simulink model "sg_lens_correct"  (Simulink 8.2)
settings: Solver=VariableStepDiscrete  StartTime=0.0  StopTime=7*Npxl  RelTol=1e-3
values from neighbouring files (symbols this model uses):
  ImgStrmIn = ImgDist'    [tb_lens_correct.m]
  ImgX = SizeI(2)    [tb_lens_correct.m]
  Npxl = ImgY * ImgX    [tb_lens_correct.m]
libraries: xbsIndex_r4 x10, dspsrcs4 x3
settings Model: Creator=sps  LastModifiedBy=tawassne
settings OptimizationCC: InitFltsAndDblsToZero=on
settings DebuggingCC: SaveWithParameterizedLinksMsg=none  SignalResolutionControl=TryResolveAllWithWarning  SolverPrmCheckMsg=none  MultiTaskDSMMsg=warning  MultiTaskCondExecSysMsg=none
settings RTWCC: IncludeERTFirstTime=on
settings GRTTargetCC: TargetFcnLib=ansi_tfl_tmw.mat

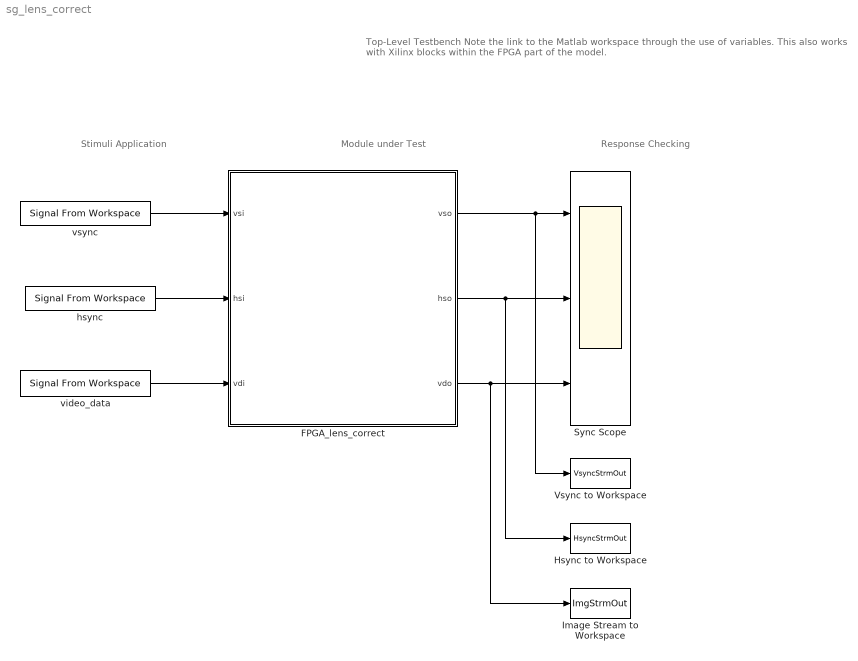
== system sg_lens_correct ==
  note: Top-Level Testbench
      | Note the link to the Matlab workspace through the use of variables.
      | This also works with Xilinx blocks within the FPGA part of the model.
  note: Stimuli Application
  note: Response Checking
  note: Module under Test
  FPGA_lens_correct : Subsystem
  Hsync to Workspace : ToWorkspace  VariableName=HsyncStrmOut  SampleTime=-1
      settings: MaxDataPoints=2*Npxl
  Image Stream to Workspace : ToWorkspace  VariableName=ImgStrmOut  SampleTime=-1
      settings: MaxDataPoints=2*Npxl
  Sync Scope : Scope  NumInputPorts=3
      settings: YMin=-5~-5~-5  YMax=5~5~5
  Vsync to Workspace : ToWorkspace  VariableName=VsyncStrmOut  SampleTime=-1
      settings: MaxDataPoints=2*Npxl
  hsync : dspsrcs4/Signal From Workspace  X=[ zeros(1,ImgX-1) 1 ]  Ts=1  nsamps=1  OutputAfterFinalValue=Cyclic repetition  ignoreOrWarnInputAndFrameLengths=off
  video_data : dspsrcs4/Signal From Workspace  X=[ ImgStrmIn(:) ]  Ts=1  nsamps=1  OutputAfterFinalValue=Cyclic repetition  ignoreOrWarnInputAndFrameLengths=off
  vsync : dspsrcs4/Signal From Workspace  X=[ zeros(1,Npxl-1) 1 ]  Ts=1  nsamps=1  OutputAfterFinalValue=Cyclic repetition  ignoreOrWarnInputAndFrameLengths=off
  wires:
  vsync/1 -> FPGA_lens_correct/1(vsi)
  hsync/1 -> FPGA_lens_correct/2(hsi)
  video_data/1 -> FPGA_lens_correct/3(vdi)
  FPGA_lens_correct/1(vso) -> Sync Scope/1, Vsync to Workspace/1
  FPGA_lens_correct/2(hso) -> Sync Scope/2, Hsync to Workspace/1
  FPGA_lens_correct/3(vdo) -> Sync Scope/3, Image Stream to Workspace/1

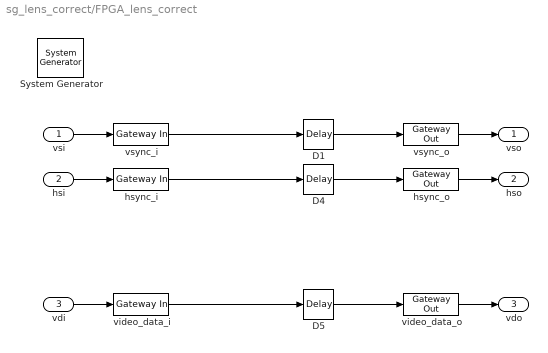
== system sg_lens_correct/FPGA_lens_correct ==
  vsi : Inport
  hsi : Inport  Port=2
  vdi : Inport  Port=3
  " System Generator" : xbsIndex_r4/ System Generator  Tag=genX  xilinxfamily=spartan6  part=xc6slx150t  speed=-3  package=fgg676  synthesis_tool=XST  clock_wrapper=Clock Enables  directory=./sg_gamma_s6  proj_type=Project Navigator  Synth_file=XST Defaults  Impl_file=ISE Defaults  testbench=off  simulink_period=1  sysclk_period=10  dcm_input_clock_period=10  incr_netlist=off  trim_vbits=Everywhere in SubSystem  dbl_ovrd=According to Block Masks  core_generation=According to Block Masks  run_coregen=off  deprecated_control=off  eval_field=0  block_type=sysgen
      settings: block_version=11.4
  D1 : xbsIndex_r4/Delay  rst=off  infoeditControl=Selection of Reset will increase slice count due to use of real FFs and instead of SRLs  en=off  latency=1  dbl_ovrd=off  reg_retiming=off  block_type=delay
  D4 : xbsIndex_r4/Delay  rst=off  infoeditControl=Selection of Reset will increase slice count due to use of real FFs and instead of SRLs  en=off  latency=1  dbl_ovrd=off  reg_retiming=off  block_type=delay
  D5 : xbsIndex_r4/Delay  rst=off  infoeditControl=Selection of Reset will increase slice count due to use of real FFs and instead of SRLs  en=off  latency=1  dbl_ovrd=off  reg_retiming=off  block_type=delay
  hsync_i : xbsIndex_r4/Gateway In  gui_display_data_type=Fixed-point  arith_type=Boolean  n_bits=1  bin_pt=0  preci_type=Single  exp_width=8  frac_width=24  quantization="Round  (unbiased: +/- Inf)"  overflow=Saturate  period=1  dbl_ovrd=off  timing_constraint=None  locs_specified=off  LOCs={}  hdl_port=on  block_type=gatewayin
      settings: infoedit="Gateway in block.  Converts inputs of type Simulink integer, double and fixed point to  Xilinx fixed point type.<br><br>Hardware notes:  In hardware these blocks become top level input ports."  xl_area=[0, 0, 0, 0, 0, 0, 0]  block_version=VER_STRING_GOES_HERE
  hsync_o : xbsIndex_r4/Gateway Out  hdl_port=on  timing_constraint=None  locs_specified=off  LOCs={}  block_type=gatewayout
      settings: infoedit="Gateway out block.  Converts Xilinx fixed point inputs into ouputs of type Simulink integer, double, or fixed point.<P><P>Hardware notes:  In hardware these blocks become top level output ports or are discarded, depending on how they are configured."  xl_area=[0, 0, 0, 0, 0, 0, 0]  block_version=VER_STRING_GOES_HERE
  video_data_i : xbsIndex_r4/Gateway In  gui_display_data_type=Fixed-point  arith_type=Unsigned  n_bits=8  bin_pt=0  preci_type=Single  exp_width=8  frac_width=24  quantization="Round  (unbiased: +/- Inf)"  overflow=Saturate  period=1  dbl_ovrd=off  timing_constraint=None  locs_specified=off  LOCs={}  hdl_port=on  block_type=gatewayin
      settings: infoedit="Gateway in block.  Converts inputs of type Simulink integer, double and fixed point to  Xilinx fixed point type.<br><br>Hardware notes:  In hardware these blocks become top level input ports."  xl_area=[0, 0, 0, 0, 0, 0, 0]  block_version=VER_STRING_GOES_HERE
  video_data_o : xbsIndex_r4/Gateway Out  hdl_port=on  timing_constraint=None  locs_specified=off  LOCs={}  block_type=gatewayout
      settings: infoedit="Gateway out block.  Converts Xilinx fixed point inputs into ouputs of type Simulink integer, double, or fixed point.<P><P>Hardware notes:  In hardware these blocks become top level output ports or are discarded, depending on how they are configured."  xl_area=[0, 0, 0, 0, 0, 0, 0]  block_version=VER_STRING_GOES_HERE
  vsync_i : xbsIndex_r4/Gateway In  gui_display_data_type=Fixed-point  arith_type=Boolean  n_bits=1  bin_pt=0  preci_type=Single  exp_width=8  frac_width=24  quantization="Round  (unbiased: +/- Inf)"  overflow=Saturate  period=1  dbl_ovrd=off  timing_constraint=None  locs_specified=off  LOCs={}  hdl_port=on  block_type=gatewayin
      settings: infoedit="Gateway in block.  Converts inputs of type Simulink integer, double and fixed point to  Xilinx fixed point type.<br><br>Hardware notes:  In hardware these blocks become top level input ports."  xl_area=[0, 0, 0, 0, 0, 0, 0]  block_version=VER_STRING_GOES_HERE
  vsync_o : xbsIndex_r4/Gateway Out  hdl_port=on  timing_constraint=None  locs_specified=off  LOCs={}  block_type=gatewayout
      settings: infoedit="Gateway out block.  Converts Xilinx fixed point inputs into ouputs of type Simulink integer, double, or fixed point.<P><P>Hardware notes:  In hardware these blocks become top level output ports or are discarded, depending on how they are configured."  xl_area=[0, 0, 0, 0, 0, 0, 0]  block_version=VER_STRING_GOES_HERE
  vso : Outport
  hso : Outport  Port=2
  vdo : Outport  Port=3
  wires:
  vdi/1 -> video_data_i/1
  video_data_o/1 -> vdo/1
  vsi/1 -> vsync_i/1
  hsi/1 -> hsync_i/1
  vsync_o/1 -> vso/1
  hsync_o/1 -> hso/1
  vsync_i/1 -> D1/1
  hsync_i/1 -> D4/1
  video_data_i/1 -> D5/1
  D1/1 -> vsync_o/1
  D4/1 -> hsync_o/1
  D5/1 -> video_data_o/1
